simulink model "Calibration_2020a"  (R2020a)
settings: Solver=FixedStepDiscrete  StartTime=0.0  StopTime=10.0  FixedStep=0.001  RelTol=1e-3  EnableMultiTasking=on
InitFcn:
  | EcoCoder_PreCheckLic();
libraries: CoderSF_BSW_Libs x9
settings Model: Creator=timot  LastModifiedBy=Thibault NOUVELLON
settings DataIOCC: SaveFormat=Structure  SignalLoggingSaveFormat=ModelDataLogs  SaveOutput=off  SignalLogging=off  DSMLogging=off  SaveTime=off  ReturnWorkspaceOutputs=off
settings OptimizationCC: DefaultParameterBehavior=Inlined  InlineInvariantSignals=on  EnhancedBackFolding=on  StrengthReduction=on  EnableMemcpy=off  PassReuseOutputArgsAs=Individual arguments  EfficientFloat2IntCast=on  LifeSpan=1  SimCompilerOptimization=on  OptimizeBlockOrder=speed  DifferentSizesBufferReuse=on  EfficientTunableParamExpr=on
settings DebuggingCC: AlgebraicLoopMsg=none  ArtificialAlgebraicLoopMsg=none  SaveWithDisabledLinksMsg=none  SaveWithParameterizedLinksMsg=none  CheckSSInitialOutputMsg=off  UnderspecifiedInitializationDetection=Classic  SignalResolutionControl=TryResolveAll  BlockPriorityViolationMsg=error  MinStepSizeMsg=none  InheritedTsInSrcMsg=none  MultiTaskDSMMsg=none  MultiTaskCondExecSysMsg=none  MultiTaskRateTransMsg=warning  TasksWithSamePriorityMsg=none  SigSpecEnsureSampleTimeMsg=none  IntegerOverflowMsg=error  Int32ToFloatConvMsg=none  ParameterPrecisionLossMsg=none  ParameterTunabilityLossMsg=none  FixptConstOverflowMsg=error  FcnCallInpInsideContextMsg=warning  UnconnectedInputMsg=error  UnconnectedOutputMsg=error  UnconnectedLineMsg=error  FrameProcessingCompatibilityMsg=none  BusObjectLabelMismatch=none  RootOutportRequireBusObject=none  UnknownTsInhSupMsg=none  ModelReferenceDataLoggingMessage=none  OperatingPointInterfaceChecksumMismatchMsg=none  SFUnusedDataAndEventsDiag=none  SFUnexpectedBacktrackingDiag=none  SFInvalidInputDataAccessInChartInitDiag=none  SFNoUnconditionalDefaultTransitionDiag=none  SFTransitionOutsideNaturalParentDiag=none  SFUnreachableExecutionPathDiag=none  SFMachineParentedDataDiag=error
settings HardwareCC: ProdBitPerPointer=32  ProdBitPerSizeT=32  ProdBitPerPtrDiffT=32  ProdLargestAtomicInteger=Long  ProdLargestAtomicFloat=Double  ProdEndianess=BigEndian  ProdWordSize=32  ProdHWDeviceType=Freescale->MPC55xx
settings ModelReferenceCC: UpdateModelReferenceTargets=Force  ModelReferenceNumInstancesAllowed=Single  PropagateSignalLabelsOutOfModel=off
settings SFSimCC: SFSimEcho=off  MATLABDynamicMemAlloc=off
settings RTWCC: Description=Ecotrons MPC5xxx  SystemTargetFile=MPC5644A.tlc  GenerateMakefile=off  TemplateMakefile=ert_default_tmf  RTWVerbose=off  RetainRTWFile=on  RTWCompilerOptimization=on
settings CodeAppCC: IgnoreCustomStorageClasses=off  OperatorAnnotations=on  CustomSymbolStrGlobalVar=$N$M  CustomSymbolStrType=$N$M  CustomSymbolStrFcn=$N$M  CustomSymbolStrFcnArg=$N$M  CustomSymbolStrBlkIO=$N$M  CustomSymbolStrMacro=$N$M
settings STFCustomTargetCC: TargetLangStandard=C99 (ISO)  CodeReplacementLibrary=ANSI_C  UtilityFuncGeneration=Shared location  MultiwordLength=256  IncludeMdlTerminateFcn=off  CombineOutputUpdateFcns=on  SuppressErrorStatus=on  ERTCustomFileBanners=on  SupportNonFinite=off  SupportComplex=off  SupportContinuousTime=off  SupportNonInlinedSFcns=off  MATLABClassNameForMDSCustomization=Simulink.SoftwareTarget.ERTCustomization  SystemTargetFile=MPC5644A.tlc
settings ERTTargetCC: TargetLangStandard=C99 (ISO)  CodeReplacementLibrary=ANSI_C  UtilityFuncGeneration=Shared location  ParMdlRefBuildCompliant=off  CompOptLevelCompliant=off  ConcurrentExecutionCompliant=off  IncludeMdlTerminateFcn=off  SuppressErrorStatus=on  SupportNonFinite=off  SupportComplex=off  RemoveResetFunc=off  ModelStepFunctionPrototypeControlCompliant=off  CPPClassGenCompliant=off  UseToolchainInfoCompliant=off  GenerateASAP2=on  InlinedParameterPlacement=NonHierarchical  ERTCustomFileTemplate=MPC5644A_file_process.tlc  ERTFilePackagingFormat=Compact  PreserveIfCondition=on  ConvertIfToSwitch=off  PreserveExternInFcnDecls=off  SuppressUnreachableDefaultCases=off

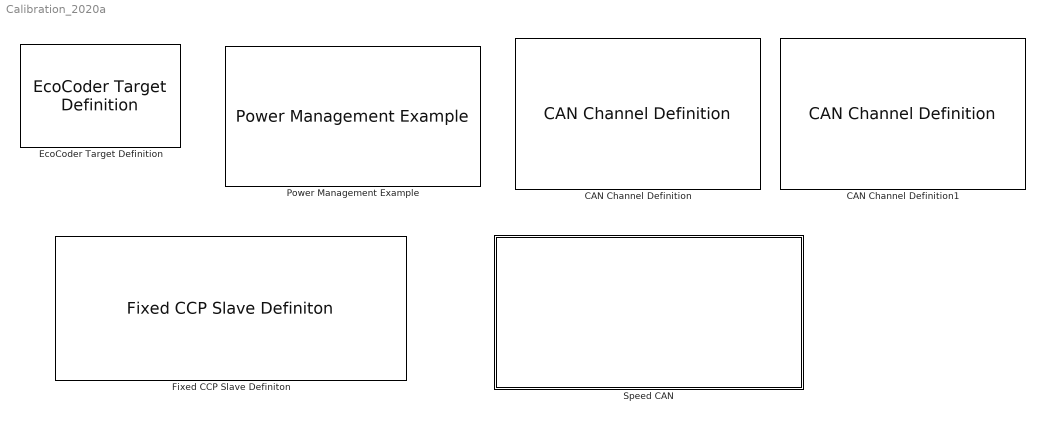
== system Calibration_2020a ==
  CAN Channel Definition : CoderSF_BSW_Libs/CAN/CAN Channel Definition  channel=CAN_B  can_en=on  can_idfilter=off  can_rxextended=off  can_rxMask=hex2dec('7ff')  can_rxID=hex2dec('100')  can_baudrateIndex=500  can_txbuffer_size=20  can_rxbuffer_size=1  can_en_fd=off  nominalSamplePoint=7500  can_baudrateIndex_data=500  fastSamplePoint=7500  canfd_txbuffer_size=5  EcoCoderBlockID=C001_CANDef
  CAN Channel Definition1 : CoderSF_BSW_Libs/CAN/CAN Channel Definition  channel=CAN_A  can_en=on  can_idfilter=off  can_rxextended=off  can_rxMask=hex2dec('7ff')  can_rxID=hex2dec('100')  can_baudrateIndex=500  can_txbuffer_size=20  can_rxbuffer_size=1  can_en_fd=off  nominalSamplePoint=7500  can_baudrateIndex_data=500  fastSamplePoint=7500  canfd_txbuffer_size=5  EcoCoderBlockID=C001_CANDef
  EcoCoder Target Definition : CoderSF_BSW_Libs/EcoCoder Target Definition  targetECU=EV2274A  EcoCoderBlockID=T001_Target  enNoTriggerCall=on  flgBlockReduction=on  flgShowDebugDisp=off  flgDisTargetOutFIleCounter=off  flgClearAllOldFiles=on  tc275_cal_len=hex2dec('00008000')  internal_flash=[hex2dec('00020000'),hex2dec('000E0000')]  cal_rom_phy=[hex2dec('00010000'),hex2dec('00002000')]  cal_ram_wp=[hex2dec('4000F000'),hex2dec('00002000')]  cal_ram_msm=[hex2dec('40000000'),hex2dec('00002000')]  var_ram_wp=[hex2dec('40002000'),hex2dec('0000D000')]  write_back_fixed_ram=[hex2dec('40011000'),hex2dec('00001000')]  write_back_unfixed_ram=[hex2dec('40012000'),hex2dec('00001000')]  stack=[hex2dec('40013000'),hex2dec('00001000')]
      settings: AttributesFormatString=Target :%<targetECU>
  Fixed CCP Slave Definiton : CoderSF_BSW_Libs/CCP/Fixed CCP Slave Definiton  ccpType=Configurable  ccp_enSet=on  ccp_disASW=on  channel=CAN_B  stationaddressSet=hex2dec('0112')  croidSet=hex2dec('100')  dtoidSet=hex2dec('101')  daqidSet=[hex2dec('101') hex2dec('101') hex2dec('101') hex2dec('102')]  daqpidSet=[hex2dec('0') hex2dec('3C') hex2dec('78') hex2dec('0')]  daqlenSet=[hex2dec('0') hex2dec('20') hex2dec('30') hex2dec('30')]  daqperSet=[5 20 100 0]  EcoCoderBlockID=C002_CCP21Conf
  Power Management Example : CoderSF_BSW_Libs/System Management Blocks/Power Management Example  Priority=1  flgKeyFromIn=off  tKeyOffDelaySet=0.5  flgResetSWEnSet=1  tDbncKeyOffFallSet=0.1  tDbncKeyOffRiseSet=0.1  facAd2VoltSet=109/27846  uKeyOffThrSet=1  uKeyOnHystSet=1  flgCANRxLiveCheckEn=0  flgEnPwrDwnFailReset=0  flgNVMEn=on  tShtDwnWait=500  flgPwrDwnByEdgeTrigger=off  EcoCoderBlockID=PME001_Def
      settings: AttributesFormatString=Priority:%<Priority>
  Speed CAN : Subsystem  Priority=2

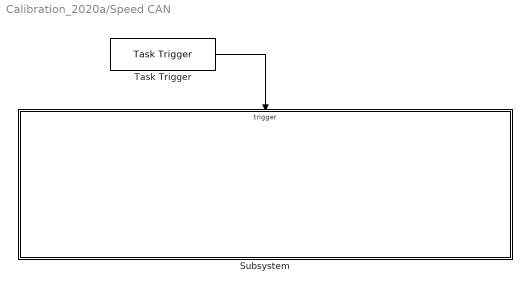
== system Calibration_2020a/Speed CAN ==
  Subsystem : Subsystem
  Task Trigger : CoderSF_BSW_Libs/Task Scheduler/Task Trigger  tasktimeIndex=Task_L100ms
  wires:
  Task Trigger/1 -> Subsystem/Trigger

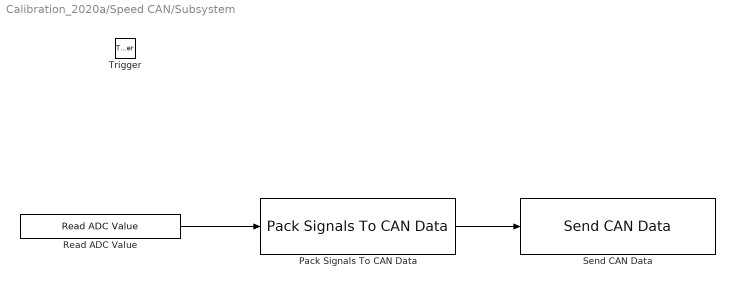
== system Calibration_2020a/Speed CAN/Subsystem ==
  Trigger : TriggerPort  TriggerType=function-call  VariantControl=Variant  PortDimensions=1
  Pack Signals To CAN Data : CoderSF_BSW_Libs/CAN/Pack Signals To CAN Data  Signal={{'test1'},[0],[8],{'uint8'},{'Intel'}}
  Read ADC Value : CoderSF_BSW_Libs/ADC/Read ADC Value  channel=19
  Send CAN Data : CoderSF_BSW_Libs/CAN/Send CAN Data  channel=CAN_A  txlen=2  txid=hex2dec('101')  frametype=Standard(11-bit ID)  showerror=off
  wires:
  Pack Signals To CAN Data/1 -> Send CAN Data/1
  Read ADC Value/1 -> Pack Signals To CAN Data/1
